simulink model "PP_simulink_control_client_2"  (R2024b)
settings: Solver=ode4  StartTime=0.0  StopTime=60  FixedStep=0.05  RelTol=1e-3
values from neighbouring files (symbols this model uses):
  Ac = LinSystem.Ac    [PP_matlab_client_Otacky.m]    (also in PP_matlab_client_Sily.m; PP_sync_matlab_client.m)
  b_moment = 5.4e-6    (= 5.4e-06)    [PP_matlab_client_Otacky.m]    (also in PP_matlab_client_Sily.m; PP_sync_matlab_client.m)
  Bc = LinSystem.Bc    [PP_matlab_client_Otacky.m]    (also in PP_matlab_client_Sily.m; PP_sync_matlab_client.m)
  k_thrust = 2.3e-3    (= 0.0023)    [PP_matlab_client_Otacky.m]    (also in PP_matlab_client_Sily.m; PP_sync_matlab_client.m)
  l = 0.2051    [PP_matlab_client_Otacky.m]    (also in PP_matlab_client_Sily.m; PP_sync_matlab_client.m)
  L_obs = place(Ac', Cc', poles_obs)'    [PP_koeficienty.m]
  Us_p = [(M+m)*g; 0; 0; 0]    [PP_matlab_client_Sily.m]    (also in PP_sync_matlab_client.m)
undefined symbols (not defined in the file or in its folder): ki, kp
libraries: simulink_extras x5
settings Model: Creator=yaozhong.zhang  LastModifiedBy=Admin
settings DebuggingCC: UnconnectedInputMsg=warning  UnconnectedOutputMsg=warning  UnconnectedLineMsg=warning
settings ModelReferenceCC: EnableRefExpFcnMdlSchedulingChecks=on
settings RTWCC: GPUComputeCapability=3.5

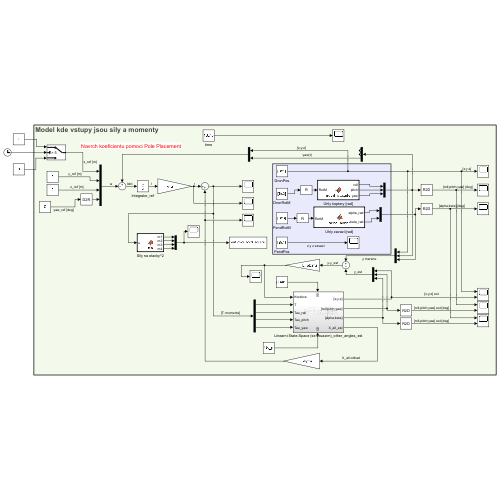
[thumbnail: Simulink's stored preview of the top-level diagram]
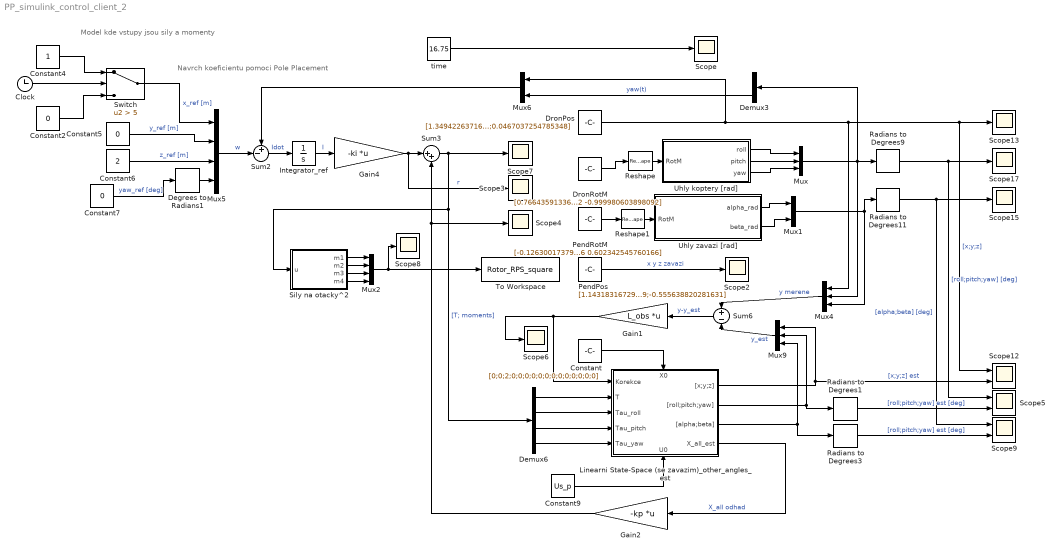
== system PP_simulink_control_client_2 ==
  note: Model kde vstupy jsou sily a momenty
  note: Navrch koeficientu pomoci Pole Placement
  Clock : Clock
  Constant : Constant  Value=[0;0;2;0;0;0;0;0;0;0;0;0;0;0;0;0]
  Constant2 : Constant  Value=0
  Constant4 : Constant
  Constant5 : Constant  Value=0
  Constant6 : Constant  Value=2
  Constant7 : Constant  Value=0
  Constant9 : Constant  Value=Us_p
  Degrees to Radians1 : simulink_extras/Transformations/Degrees to Radians
  Demux3 : Demux  Outputs=3
  Demux6 : Demux
  DronPos : Constant  Value=[1.34942263716032;-3.23979284246577;0.0467037254785348]  SampleTime=-1
  DronRotM : Constant  Value=[0.766435913366618 0.642320435575919 0.000669883153213676;0.642311444500542 -0.766418727054251 -0.0061921792746031;-0.00346395229526613 0.00517618219384752 -0.999980603898092]  SampleTime=-1
  Gain1 : Gain  Gain=L_obs  Multiplication=Matrix(K*u)
  Gain2 : Gain  Gain=-kp  Multiplication=Matrix(K*u)
  Gain4 : Gain  Gain=-ki  Multiplication=Matrix(K*u)
  Integrator_ref : Integrator  InitialCondition=[0.763403066640312;0.049470978779298;-4.03562730231744;0.245701408942988]
  Linearni State-Space (se zavazim)_other_angles_est : Subsystem
      settings: PortSchema="{\"entries\":[{\"content\":{\"sides\":[{\"content\":{\"connectorIds\":[\"In1\",\"In2\",\"In3\",\"In4\",\"In5\"]},\"type\":\"ConnectorPlacement.EquallySpacedRectSide\",\"uuid\":\"a4429057-2b47-419f-9dfc-835e85a09133\"},{\"content\":{\"connectorIds\":[\"Out1\",\"Out2\",\"Out3\",\"Out4\"],\"side\":\"RIGHT\"},\"type\":\"ConnectorPlacement.EquallySpacedRectSide\",\"uuid\":\"1ad51c71-1e63-4d5a-846d-5c19a5472817\"},{\"content\":{\"connectorIds\":[\"In6\"],\"side\":\"TOP\"},\"type\":\"ConnectorPlacement.EquallySpacedRectSide\",\"uuid\":\"31d767be-76b5-41bf-92d8-105ca7d2a947\"},{\"content\":{\"connectorIds\":[\"In7\"],\"side\":\"BOTTOM\"},\"type\":\"ConnectorPlacement.EquallySpacedRectSide\",\"uuid\":\"9694baa9-ade4-493b-8aff-3f67e2f95857\"}]},\"type\":\"ConnectorPlacement.EquallySpacedConnector\",\"uuid\":\"786fba35-a58c-42dc-a308-7daf752dfb0b\"}],\"packageUris\":[\"http://schema.mathworks.com/mf0/Connector/R2020b\"],\"version\":\"1.0\"}"
  Mux : Mux  Inputs=3
  Mux1 : Mux  Inputs=2
  Mux2 : Mux
  Mux4 : Mux  Inputs=3
  Mux5 : Mux
  Mux6 : Mux  Inputs=2
  Mux9 : Mux  Inputs=3
  PendPos : Constant  Value=[1.14318316729766;-2.46865813397579;-0.555638820281631]  SampleTime=-1
  PendRotM : Constant  Value=[-0.126300173799986 -0.970316209886684 0.206239469862661;0.589448168984251 -0.240628588166875 -0.771134708489981;0.797871620111409 0.0241730301773416 0.602342545760166]  SampleTime=-1
  Radians to Degrees{1,3,9,11} (4 alike) : simulink_extras/Transformations/Radians to Degrees
  Reshape : Reshape  OutputDimensionality=Customize  OutputDimensions=[3,3]
  Reshape1 : Reshape  OutputDimensionality=Customize  OutputDimensions=[3,3]
  Scope{,2..4,6..8,13,15,17} (10 alike) : Scope
  Scope12 : Scope  NumInputPorts=2
  Scope5 : Scope  NumInputPorts=2
  Scope9 : Scope  NumInputPorts=2
  Sily na otacky^2 : MATLAB Function  TreatAsAtomicUnit=on
  Sum2 : Sum  Inputs=+-|
  Sum3 : Sum  Inputs=|++
  Sum6 : Sum  Inputs=+|-
  Switch : Switch  Criteria=u2 > Threshold  Threshold=5  SaturateOnIntegerOverflow=off  InputSameDT=off
  To Workspace : ToWorkspace  VariableName=Rotor_RPS_square  SampleTime=-1
  Uhly koptery [rad] : MATLAB Function  TreatAsAtomicUnit=on
  Uhly zavazi [rad] : MATLAB Function  TreatAsAtomicUnit=on
  time : Constant  Value=16.75  SampleTime=-1
  wires:
  DronRotM/1 -> Reshape/1
  Uhly koptery [rad]/2(pitch) -> Mux/2
  Uhly koptery [rad]/1(roll) -> Mux/1
  Uhly koptery [rad]/3(yaw) -> Mux/3
  PendPos/1 -> Scope2/1  "x y z zavazi"
  Reshape/1 -> Uhly koptery [rad]/1(RotM)
  PendRotM/1 -> Reshape1/1
  Reshape1/1 -> Uhly zavazi [rad]/1(RotM)
  Uhly zavazi [rad]/1(alpha_rad) -> Mux1/1
  Uhly zavazi [rad]/2(beta_rad) -> Mux1/2
  time/1 -> Scope/1
  Mux6/1 -> Sum2/1
  Gain2/1 -> Sum3/2, Scope4/1
  Sum2/1 -> Integrator_ref/1  "Idot"
  Constant5/1 -> Mux5/2  "y_ref [m]"
  Constant6/1 -> Mux5/3  "z_ref [m]"
  Mux/1 -> Demux3/1, Radians to Degrees9/1, Mux4/2
  Switch/1 -> Mux5/1  "x_ref [m]"
  Integrator_ref/1 -> Gain4/1  "I"
  Demux3/3 -> Mux6/2  "yaw(t)"
  Degrees to Radians1/1 -> Mux5/4
  Constant7/1 -> Degrees to Radians1/1  "yaw_ref [deg]"
  Mux5/1 -> Sum2/2  "w"
  Mux1/1 -> Mux4/3, Radians to Degrees11/1
  Gain4/1 -> Scope3/1, Sum3/1  "r"
  Sum3/1 -> Scope7/1, Sily na otacky^2/1(u), Demux6/1  "[T; moments]"
  Linearni State-Space (se zavazim)_other_angles_est/1("[x;y;z]") -> Scope12/2, Mux9/1  "[x;y;z] est"
  Gain1/1 -> Linearni State-Space (se zavazim)_other_angles_est/1(Korekce), Scope6/1
  Radians to Degrees9/1 -> Scope5/1, Scope17/1  "[roll;pitch;yaw] [deg]"
  Linearni State-Space (se zavazim)_other_angles_est/3("[alpha;beta]") -> Mux9/3, Radians to Degrees3/1
  Linearni State-Space (se zavazim)_other_angles_est/2("[roll;pitch;yaw]") -> Mux9/2, Radians to Degrees1/1
  Radians to Degrees11/1 -> Scope9/1, Scope15/1  "[alpha;beta] [deg]"
  Radians to Degrees1/1 -> Scope5/2  "[roll;pitch;yaw] est [deg]"
  Demux6/1 -> Linearni State-Space (se zavazim)_other_angles_est/2(T)
  Mux4/1 -> Sum6/1  "y merene"
  DronPos/1 -> Scope12/1, Scope13/1, Mux4/1, Mux6/1  "[x;y;z]"
  Demux6/2 -> Linearni State-Space (se zavazim)_other_angles_est/3(Tau_roll)
  Linearni State-Space (se zavazim)_other_angles_est/4(X_all_est) -> Gain2/1  "X_all odhad"
  Demux6/4 -> Linearni State-Space (se zavazim)_other_angles_est/5(Tau_yaw)
  Mux9/1 -> Sum6/2  "y_est"
  Demux6/3 -> Linearni State-Space (se zavazim)_other_angles_est/4(Tau_pitch)
  Radians to Degrees3/1 -> Scope9/2  "[roll;pitch;yaw] est [deg]"
  Sum6/1 -> Gain1/1  "y-y_est"
  Constant9/1 -> Linearni State-Space (se zavazim)_other_angles_est/7(U0)
  Constant/1 -> Linearni State-Space (se zavazim)_other_angles_est/6(X0)
  Constant4/1 -> Switch/1
  Clock/1 -> Switch/2
  Constant2/1 -> Switch/3
  Sily na otacky^2/2(m2) -> Mux2/2
  Mux2/1 -> Scope8/1, To Workspace/1
  Sily na otacky^2/1(m1) -> Mux2/1
  Sily na otacky^2/3(m3) -> Mux2/3
  Sily na otacky^2/4(m4) -> Mux2/4

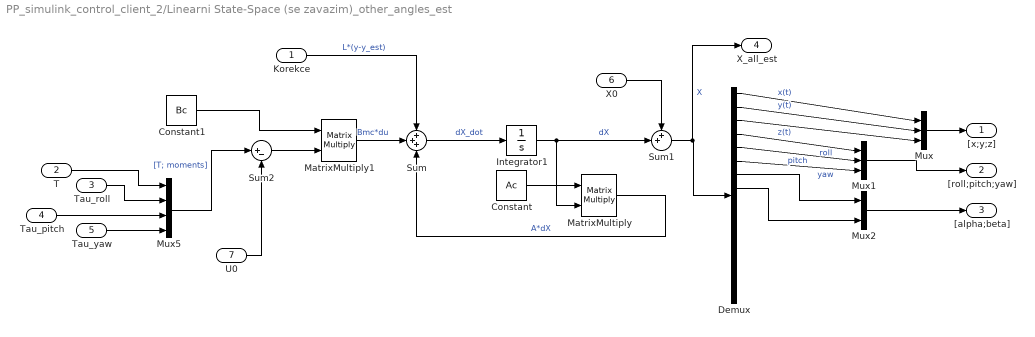
== system PP_simulink_control_client_2/Linearni State-Space (se zavazim)_other_angles_est ==
  Korekce : Inport
  T : Inport  Port=2
  Tau_roll : Inport  Port=3
  Tau_pitch : Inport  Port=4
  Tau_yaw : Inport  Port=5
  X0 : Inport  Port=6
  U0 : Inport  Port=7
  Constant : Constant  Value=Ac
  Constant1 : Constant  Value=Bc
  Demux : Demux  Outputs=16
  Integrator1 : Integrator  InitialCondition=[0;0;0;0;0;0;0;0;0;0;0;0;0;0;0;0]
  MatrixMultiply : Product  Multiplication=Matrix(*)
  MatrixMultiply1 : Product  Multiplication=Matrix(*)
  Mux : Mux  Inputs=3
  Mux1 : Mux  Inputs=3
  Mux2 : Mux  Inputs=2
  Mux5 : Mux
  Sum : Sum  Inputs=+++
  Sum1 : Sum  Inputs=++|
  Sum2 : Sum  Inputs=|+-
  "[x;y;z]" : Outport
  "[roll;pitch;yaw]" : Outport  Port=2
  "[alpha;beta]" : Outport  Port=3
  X_all_est : Outport  Port=4
  wires:
  Constant/1 -> MatrixMultiply/1
  Integrator1/1 -> Sum1/2, MatrixMultiply/2  "dX"
  Demux/1 -> Mux/1  "x(t)"
  Demux/2 -> Mux/2  "y(t)"
  Demux/3 -> Mux/3  "z(t)"
  Mux/1 -> "[x;y;z]"/1
  Demux/4 -> Mux1/1  "roll"
  Demux/5 -> Mux1/2  "pitch"
  Demux/6 -> Mux1/3  "yaw"
  Mux1/1 -> "[roll;pitch;yaw]"/1
  Sum/1 -> Integrator1/1  "dX_dot"
  MatrixMultiply1/1 -> Sum/2  "Bmc*du"
  MatrixMultiply/1 -> Sum/3  "A*dX"
  Constant1/1 -> MatrixMultiply1/1
  Sum1/1 -> X_all_est/1, Demux/1  "X"
  Sum2/1 -> MatrixMultiply1/2
  Mux2/1 -> "[alpha;beta]"/1
  Demux/7 -> Mux2/1
  Demux/8 -> Mux2/2
  Mux5/1 -> Sum2/1  "[T; moments]"
  Korekce/1 -> Sum/1  "L*(y-y_est)"
  Tau_yaw/1 -> Mux5/4
  T/1 -> Mux5/1
  Tau_pitch/1 -> Mux5/3
  Tau_roll/1 -> Mux5/2
  X0/1 -> Sum1/1
  U0/1 -> Sum2/2

== matlab function PP_simulink_control_client_2/Uhly zavazi [rad] ==
  data: RotM input; alpha_rad output; beta_rad output
function [alpha_rad, beta_rad] = pend_orient(RotM)
% Расчет углов альфа и бета маятника

% Вектор маятника
rope_vector = RotM * [0; 0; -1];

% Расчет угла альфа
rope_vector_xz = rope_vector([1, 3]); % Компоненты x и z
z_axis = [0; -1];
cos_alpha = dot(rope_vector_xz, z_axis) / (norm(rope_vector_xz) * norm(z_axis));
cos_alpha = max(-1, min(1, cos_alpha)); % Ограничиваем в диапазоне [-1, 1]
alpha = acos(cos_alpha);
if rope_vector(1) < 0
    alpha = -alpha;
end

% Расчет угла бета
rope_vector_xz_3 = [rope_vector(1); 0; rope_vector(3)];
cos_beta = dot(rope_vector, rope_vector_xz_3) / (norm(rope_vector) * norm(rope_vector_xz_3));
cos_beta = max(-1, min(1, cos_beta)); % Ограничиваем в диапазоне [-1, 1]
beta = acos(cos_beta);
if rope_vector(2) < 0
    beta = -beta;
end

% Округляем до 5 знаков после запятой
% alpha_rad = round(alpha, 5); %[rad]
% beta_rad = round(beta, 5); %[rad]
alpha_rad = alpha;
beta_rad = beta;

== matlab function PP_simulink_control_client_2/Sily na otacky^2 ==
  data: u input; m1 output; m2 output; m3 output; m4 output; b_moment parameter; k_thrust parameter; l parameter
function [m1, m2, m3, m4]= fcn(u, b_moment, k_thrust, l)

T = u(1);
Tau_phi = u(2);
Tau_theta = u(3);
Tau_psi = u(4);

m1 = ( (Tau_phi*b_moment - Tau_theta*b_moment + l*T*b_moment + l*Tau_psi*k_thrust)/(4*l*b_moment*k_thrust));
m2 = ( (-Tau_theta*b_moment - Tau_phi*b_moment + l*T*b_moment - l*Tau_psi*k_thrust)/(4*l*b_moment*k_thrust));
m3 = ( (Tau_theta*b_moment - Tau_phi*b_moment + l*T*b_moment + l*Tau_psi*k_thrust)/(4*l*b_moment*k_thrust));
m4 = ( (Tau_phi*b_moment + Tau_theta*b_moment + l*T*b_moment - l*Tau_psi*k_thrust)/(4*l*b_moment*k_thrust));

== matlab function PP_simulink_control_client_2/Uhly koptery [rad] ==
  data: RotM input; roll output; pitch output; yaw output
function [roll, pitch, yaw] = quad_attitude(RotM)
% matice rotace koptery z Python, vuci svetu!!!
% rotm2eul prevadi na Eulerove uhly
radians = rotm2eul(RotM, 'ZYX'); % pouzivam poradi ZYX

% roll = kolem x, pitch = kolem y, yaw = kolem z
yaw = radians(1);
pitch = radians(2);
roll = radians(3);
end
